simulink library "PlantLibrary"  (R2016b)
settings: Solver=VariableStepAuto  StartTime=0.0  StopTime=10.0  RelTol=1e-3
values from neighbouring files (symbols this model uses):
  amp2mAmp = 1000    [PlantParams.m]
  coilL = 0.125    [PlantParams.m]
  coilMaxI = 0.9*amp2mAmp*Vs/coilR    (= 1800)    [PlantParams.m]
  coilMinI = 0.2*amp2mAmp*Vs/coilR    (= 400)    [PlantParams.m]
  coilR = 6    [PlantParams.m]
  fs = 100    [PlantParams.m]
  maxFlowRate = maxFlowRate*1    (= 16)    [PlantParams.m]
  reducer_ex = 0.01    [PlantParams.m]
  reducer_rt = 0.01    [PlantParams.m]
  strokeLegnth = 500    [PlantParams.m]
  Vs = 12    [PlantParams.m]
undefined symbols (not defined in the file or in its folder): DiscIntNeverNeededParam
undefined symbols (not defined in the file): dampeningFL, extendRateFL, retractRateFL
libraries: PlantLibrary x19, simulink x3, HighClearance_library x1
settings Model: Creator=lemaya  LastModifiedBy=lemaya

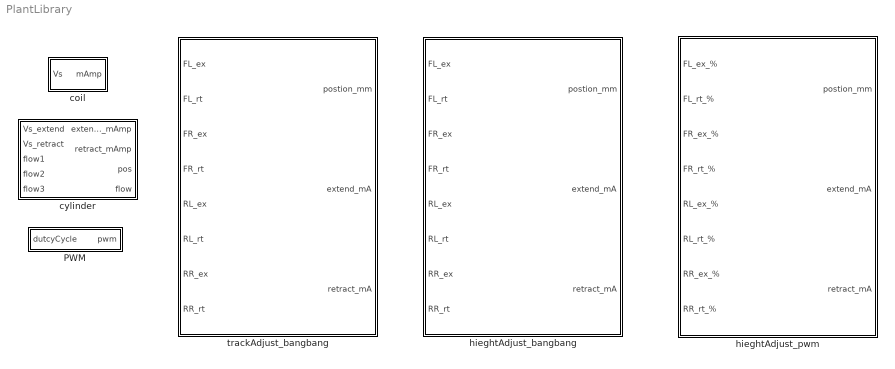
== system PlantLibrary ==
  PWM : Subsystem  TreatAsAtomicUnit=on
  coil : Subsystem
  cylinder : Subsystem  mask{dampening=dampeningFL, extendRate=extendRateFL, retractRate=retractRateFL}
      mask prompts: dampening "Dampening coefficient:"; extendRate "Extend Rate [mm/sec]:"; retractRate "Retract Rate [mm/sec]:"
  hieghtAdjust_bangbang : Subsystem
  hieghtAdjust_pwm : Subsystem
  trackAdjust_bangbang : Subsystem

== system PlantLibrary/PWM ==
  dutcyCycle : Inport
  Data Type Conversion : DataTypeConversion  OutDataTypeStr=single
  Relational Operator : RelationalOperator  Operator=>  OutDataTypeStr=boolean  RndMeth=Simplest
  freq : simulink/Sources/Repeating Sequence  rep_seq_t=[0 1/fs]  rep_seq_y=[0 100]
  pwm : Outport
  wires:
  freq/1 -> Relational Operator/2  "Hz"
  Relational Operator/1 -> Data Type Conversion/1
  dutcyCycle/1 -> Relational Operator/1  "%"
  Data Type Conversion/1 -> pwm/1

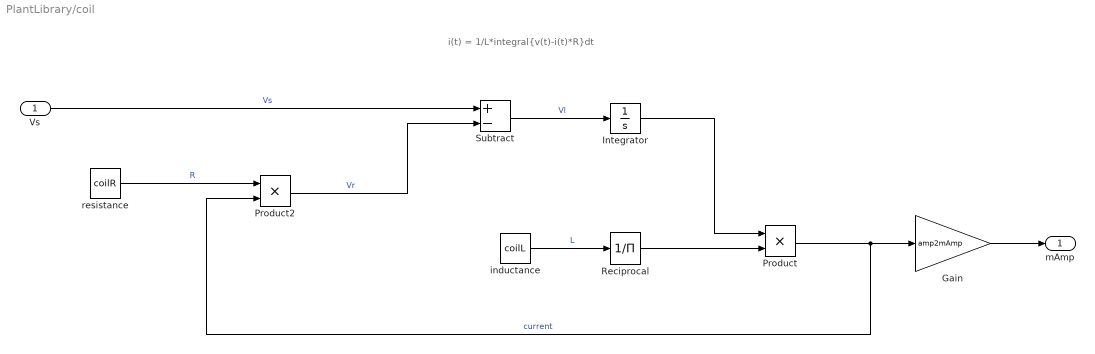
== system PlantLibrary/coil ==
  note: i(t) = 1/L*integral{v(t)-i(t)*R}dt
  Vs : Inport
  Gain : Gain  Gain=amp2mAmp  OutDataTypeStr=single
  Integrator : Integrator
  Product : Product  OutDataTypeStr=single  SaturateOnIntegerOverflow=on
  Product2 : Product  OutDataTypeStr=single  SaturateOnIntegerOverflow=on
  Reciprocal : Product  Inputs=/  SaturateOnIntegerOverflow=on  RndMeth=Zero
  Subtract : Sum  Inputs=+-  OutDataTypeStr=Inherit: Inherit via back propagation  SaturateOnIntegerOverflow=on
  inductance : Constant  Value=coilL  OutDataTypeStr=single
  resistance : Constant  Value=coilR  OutDataTypeStr=single
  mAmp : Outport
  wires:
  Gain/1 -> mAmp/1
  Vs/1 -> Subtract/1  "Vs"
  inductance/1 -> Reciprocal/1  "L"
  Subtract/1 -> Integrator/1  "Vl"
  resistance/1 -> Product2/1  "R"
  Product2/1 -> Subtract/2  "Vr"
  Integrator/1 -> Product/1
  Reciprocal/1 -> Product/2
  Product/1 -> Gain/1, Product2/2  "current"

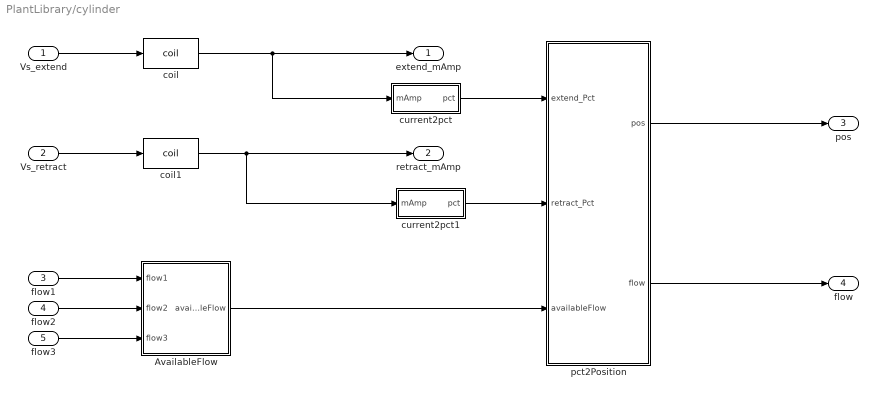
== system PlantLibrary/cylinder ==
  Vs_extend : Inport
  Vs_retract : Inport  Port=2
  flow1 : Inport  Port=3
  flow2 : Inport  Port=4
  flow3 : Inport  Port=5
  AvailableFlow : Subsystem
  coil : PlantLibrary/coil
  coil1 : PlantLibrary/coil
  current2pct : Subsystem
  current2pct1 : Subsystem
  pct2Position : Subsystem
  extend_mAmp : Outport
  retract_mAmp : Outport  Port=2
  pos : Outport  Port=3
  flow : Outport  Port=4
  wires:
  AvailableFlow/1(availableFlow) -> pct2Position/3(availableFlow)
  flow3/1 -> AvailableFlow/3(flow3)
  flow2/1 -> AvailableFlow/2(flow2)
  flow1/1 -> AvailableFlow/1(flow1)
  pct2Position/2(flow) -> flow/1
  pct2Position/1(pos) -> pos/1
  current2pct1/1(pct) -> pct2Position/2(retract_Pct)
  current2pct/1(pct) -> pct2Position/1(extend_Pct)
  coil1/1 -> retract_mAmp/1, current2pct1/1(mAmp)
  coil/1 -> extend_mAmp/1, current2pct/1(mAmp)
  Vs_retract/1 -> coil1/1
  Vs_extend/1 -> coil/1

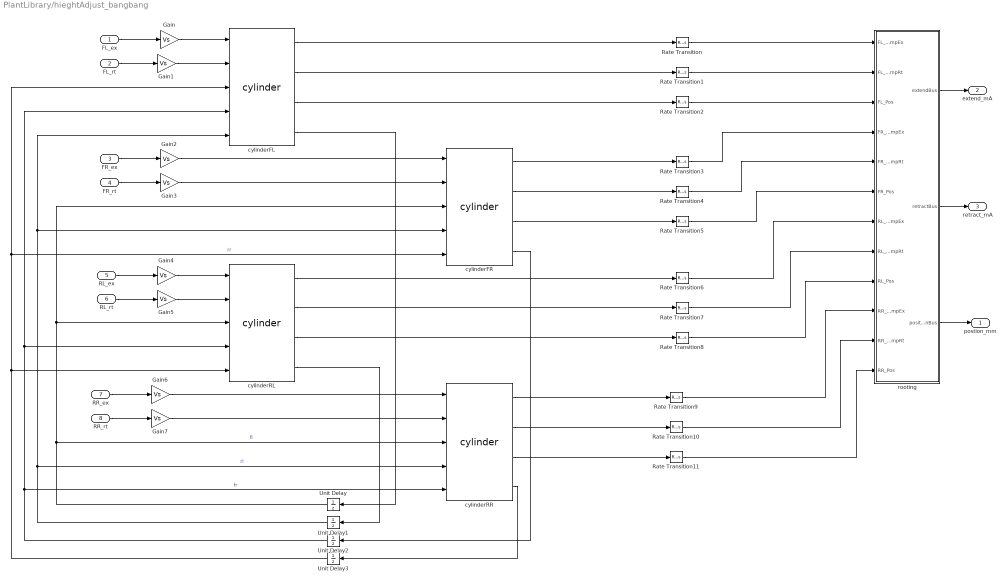
== system PlantLibrary/hieghtAdjust_bangbang ==
  FL_ex : Inport
  FL_rt : Inport  Port=2
  FR_ex : Inport  Port=3
  FR_rt : Inport  Port=4
  RL_ex : Inport  Port=5
  RL_rt : Inport  Port=6
  RR_ex : Inport  Port=7
  RR_rt : Inport  Port=8
  Gain{,1..7} (8 alike) : Gain  Gain=Vs
  Rate Transition{,1..11} (12 alike) : RateTransition
  Unit Delay{,1..3} (4 alike) : UnitDelay  SampleTime=-1
  cylinderFL : PlantLibrary/cylinder  dampening=dampeningFL  extendRate=extendRateFL  retractRate=retractRateFL
  cylinderFR : PlantLibrary/cylinder  dampening=dampeningFR  extendRate=extendRateFR  retractRate=retractRateFR
  cylinderRL : PlantLibrary/cylinder  dampening=dampeningRL  extendRate=extendRateRL  retractRate=retractRateRL
  cylinderRR : PlantLibrary/cylinder  dampening=dampeningRR  extendRate=extendRateRR  retractRate=retractRateRR
  rooting : Subsystem
  postion_mm : Outport
  extend_mA : Outport  Port=2
  retract_mA : Outport  Port=3
  wires:
  Unit Delay/1 -> cylinderRR/3, cylinderRL/3, cylinderFR/3  "fl"
  Unit Delay3/1 -> cylinderFR/5, cylinderFL/3, cylinderRL/5  "rr"
  Unit Delay2/1 -> cylinderRR/5, cylinderRL/4, cylinderFL/4  "fr"
  Unit Delay1/1 -> cylinderRR/4, cylinderFR/4, cylinderFL/5  "rl"
  cylinderRR/4 -> Unit Delay3/1
  cylinderFR/4 -> Unit Delay2/1
  cylinderRL/4 -> Unit Delay1/1
  cylinderFL/4 -> Unit Delay/1
  Gain2/1 -> cylinderFR/1
  Gain3/1 -> cylinderFR/2
  cylinderRR/3 -> Rate Transition11/1
  cylinderFR/3 -> Rate Transition5/1
  cylinderRL/3 -> Rate Transition8/1
  cylinderFL/3 -> Rate Transition2/1
  Rate Transition11/1 -> rooting/12(RR_Pos)
  Rate Transition10/1 -> rooting/11(RR_mAmpRt)
  Rate Transition9/1 -> rooting/10(RR_mAmpEx)
  Rate Transition8/1 -> rooting/9(RL_Pos)
  Rate Transition7/1 -> rooting/8(RL_mAmpRt)
  Rate Transition6/1 -> rooting/7(RL_mAmpEx)
  Rate Transition5/1 -> rooting/6(FR_Pos)
  Rate Transition4/1 -> rooting/5(FR_mAmpRt)
  Rate Transition3/1 -> rooting/4(FR_mAmpEx)
  Rate Transition2/1 -> rooting/3(FL_Pos)
  Rate Transition1/1 -> rooting/2(FL_mAmpRt)
  Rate Transition/1 -> rooting/1(FL_mAmpEx)
  Gain7/1 -> cylinderRR/2
  Gain6/1 -> cylinderRR/1
  Gain5/1 -> cylinderRL/2
  Gain4/1 -> cylinderRL/1
  Gain1/1 -> cylinderFL/2
  Gain/1 -> cylinderFL/1
  RL_rt/1 -> Gain5/1
  RR_ex/1 -> Gain6/1
  FR_rt/1 -> Gain3/1
  FR_ex/1 -> Gain2/1
  FL_ex/1 -> Gain/1
  RL_ex/1 -> Gain4/1
  RR_rt/1 -> Gain7/1
  FL_rt/1 -> Gain1/1
  rooting/1(extendBus) -> extend_mA/1
  rooting/2(retractBus) -> retract_mA/1
  rooting/3(positionBus) -> postion_mm/1
  cylinderFL/1 -> Rate Transition/1
  cylinderFL/2 -> Rate Transition1/1
  cylinderFR/1 -> Rate Transition3/1
  cylinderFR/2 -> Rate Transition4/1
  cylinderRL/1 -> Rate Transition6/1
  cylinderRL/2 -> Rate Transition7/1
  cylinderRR/1 -> Rate Transition9/1
  cylinderRR/2 -> Rate Transition10/1

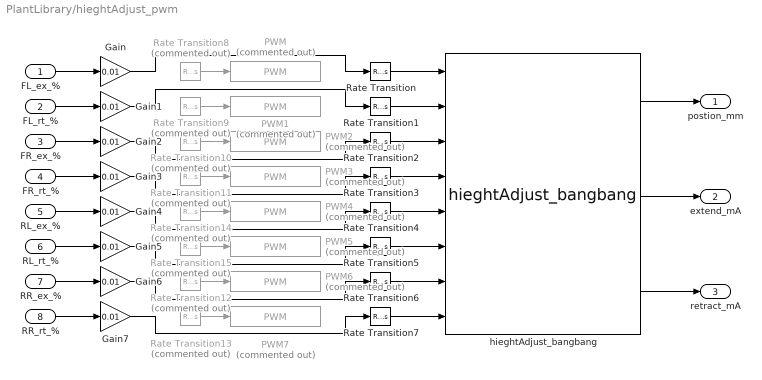
== system PlantLibrary/hieghtAdjust_pwm ==
  FL_ex_% : Inport
  FL_rt_% : Inport  Port=2
  FR_ex_% : Inport  Port=3
  FR_rt_% : Inport  Port=4
  RL_ex_% : Inport  Port=5
  RL_rt_% : Inport  Port=6
  RR_ex_% : Inport  Port=7
  RR_rt_% : Inport  Port=8
  Gain{,1..7} (8 alike) : Gain  Gain=0.01
  PWM{,1..7} (8 alike) : PlantLibrary/PWM  Commented=on
  Rate Transition{,1..7} (8 alike) : RateTransition
  Rate Transition{8..15} (8 alike) : RateTransition  Commented=on  OutPortSampleTime=0.0001
  hieghtAdjust_bangbang : PlantLibrary/hieghtAdjust_bangbang
  postion_mm : Outport
  extend_mA : Outport  Port=2
  retract_mA : Outport  Port=3
  wires:
  Gain7/1 -> Rate Transition7/1
  RR_rt_%/1 -> Gain7/1
  Gain6/1 -> Rate Transition6/1
  RR_ex_%/1 -> Gain6/1
  Gain5/1 -> Rate Transition5/1
  RL_rt_%/1 -> Gain5/1
  Gain4/1 -> Rate Transition4/1
  RL_ex_%/1 -> Gain4/1
  Gain3/1 -> Rate Transition3/1
  FR_rt_%/1 -> Gain3/1
  Gain2/1 -> Rate Transition2/1
  FR_ex_%/1 -> Gain2/1
  Gain/1 -> Rate Transition/1
  Gain1/1 -> Rate Transition1/1
  FL_rt_%/1 -> Gain1/1
  FL_ex_%/1 -> Gain/1
  Rate Transition13/1 -> PWM7/1
  Rate Transition12/1 -> PWM6/1
  Rate Transition15/1 -> PWM5/1
  Rate Transition14/1 -> PWM4/1
  Rate Transition11/1 -> PWM3/1
  Rate Transition10/1 -> PWM2/1
  Rate Transition9/1 -> PWM1/1
  Rate Transition8/1 -> PWM/1
  hieghtAdjust_bangbang/1 -> postion_mm/1
  hieghtAdjust_bangbang/3 -> retract_mA/1
  hieghtAdjust_bangbang/2 -> extend_mA/1
  Rate Transition/1 -> hieghtAdjust_bangbang/1
  Rate Transition1/1 -> hieghtAdjust_bangbang/2
  Rate Transition2/1 -> hieghtAdjust_bangbang/3
  Rate Transition3/1 -> hieghtAdjust_bangbang/4
  Rate Transition4/1 -> hieghtAdjust_bangbang/5
  Rate Transition5/1 -> hieghtAdjust_bangbang/6
  Rate Transition6/1 -> hieghtAdjust_bangbang/7
  Rate Transition7/1 -> hieghtAdjust_bangbang/8

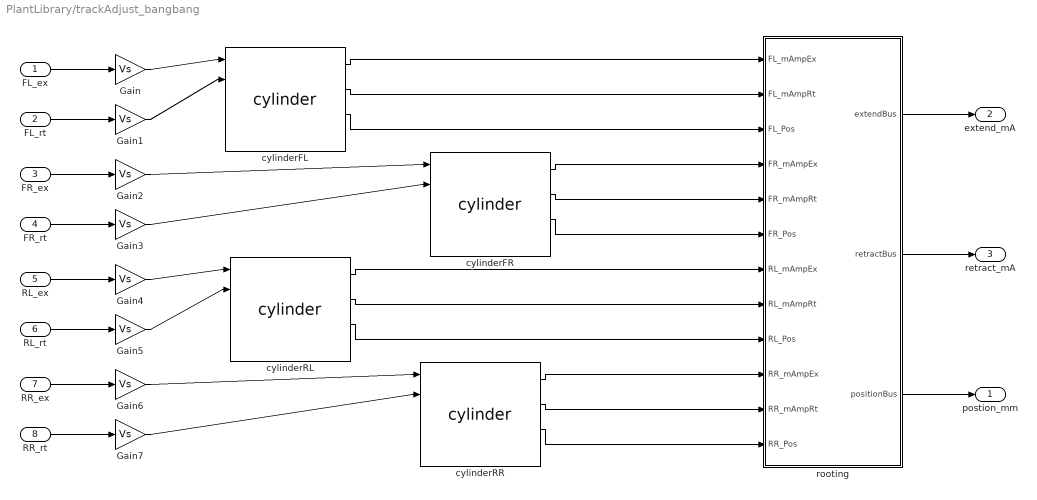
== system PlantLibrary/trackAdjust_bangbang ==
  FL_ex : Inport
  FL_rt : Inport  Port=2
  FR_ex : Inport  Port=3
  FR_rt : Inport  Port=4
  RL_ex : Inport  Port=5
  RL_rt : Inport  Port=6
  RR_ex : Inport  Port=7
  RR_rt : Inport  Port=8
  Gain{,1..7} (8 alike) : Gain  Gain=Vs
  cylinderFL : PlantLibrary/cylinder  dampening=dampening  extendRate=extendRateFL  retractRate=retractRateFL
  cylinderFR : PlantLibrary/cylinder  dampening=dampening  extendRate=extendRateFL  retractRate=retractRateFL
  cylinderRL : PlantLibrary/cylinder  dampening=dampening  extendRate=extendRateFL  retractRate=retractRateFL
  cylinderRR : PlantLibrary/cylinder  dampening=dampening  extendRate=extendRateFL  retractRate=retractRateFL
  rooting : Subsystem
  postion_mm : Outport
  extend_mA : Outport  Port=2
  retract_mA : Outport  Port=3
  wires:
  cylinderRR/3 -> rooting/12(RR_Pos)
  cylinderRR/2 -> rooting/11(RR_mAmpRt)
  cylinderRR/1 -> rooting/10(RR_mAmpEx)
  cylinderRL/3 -> rooting/9(RL_Pos)
  cylinderRL/2 -> rooting/8(RL_mAmpRt)
  cylinderRL/1 -> rooting/7(RL_mAmpEx)
  cylinderFR/3 -> rooting/6(FR_Pos)
  cylinderFR/2 -> rooting/5(FR_mAmpRt)
  cylinderFR/1 -> rooting/4(FR_mAmpEx)
  cylinderFL/3 -> rooting/3(FL_Pos)
  cylinderFL/2 -> rooting/2(FL_mAmpRt)
  cylinderFL/1 -> rooting/1(FL_mAmpEx)
  rooting/3(positionBus) -> postion_mm/1
  rooting/2(retractBus) -> retract_mA/1
  rooting/1(extendBus) -> extend_mA/1
  FL_rt/1 -> Gain1/1
  RR_rt/1 -> Gain7/1
  RL_ex/1 -> Gain4/1
  FL_ex/1 -> Gain/1
  FR_ex/1 -> Gain2/1
  FR_rt/1 -> Gain3/1
  RR_ex/1 -> Gain6/1
  RL_rt/1 -> Gain5/1
  Gain/1 -> cylinderFL/1
  Gain1/1 -> cylinderFL/2
  Gain2/1 -> cylinderFR/1
  Gain3/1 -> cylinderFR/2
  Gain4/1 -> cylinderRL/1
  Gain5/1 -> cylinderRL/2
  Gain6/1 -> cylinderRR/1
  Gain7/1 -> cylinderRR/2

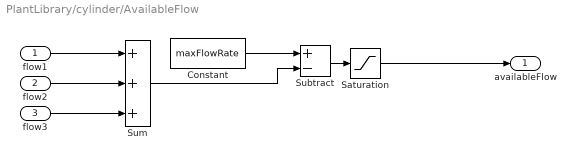
== system PlantLibrary/cylinder/AvailableFlow ==
  flow1 : Inport
  flow2 : Inport  Port=2
  flow3 : Inport  Port=3
  Constant : Constant  Value=maxFlowRate
  Saturation : Saturate  UpperLimit=0  LowerLimit=-inf
  Subtract : Sum  Inputs=+-
  Sum : Sum  Inputs=+++
  availableFlow : Outport
  wires:
  Saturation/1 -> availableFlow/1
  Subtract/1 -> Saturation/1
  Sum/1 -> Subtract/2
  flow2/1 -> Sum/2
  Constant/1 -> Subtract/1
  flow1/1 -> Sum/1
  flow3/1 -> Sum/3

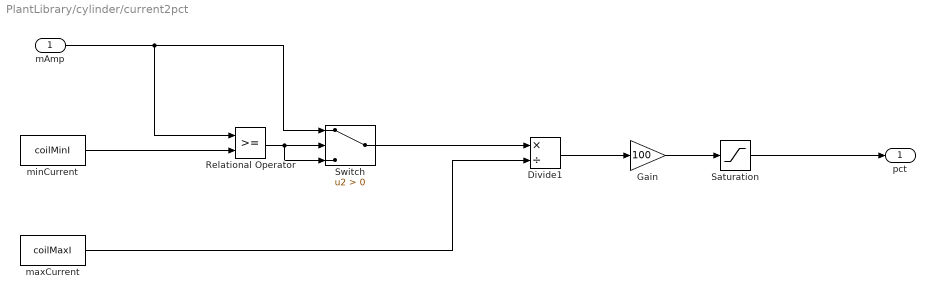
== system PlantLibrary/cylinder/current2pct ==
  mAmp : Inport
  Divide1 : Product  Inputs=*/
  Gain : Gain  Gain=100
  Relational Operator : RelationalOperator  OutDataTypeStr=boolean  RndMeth=Simplest
  Saturation : Saturate  UpperLimit=100  LowerLimit=0
  Switch : Switch  Criteria=u2 > Threshold
  maxCurrent : Constant  Value=coilMaxI
  minCurrent : Constant  Value=coilMinI
  pct : Outport
  wires:
  Gain/1 -> Saturation/1
  Saturation/1 -> pct/1
  Divide1/1 -> Gain/1
  mAmp/1 -> Switch/1, Relational Operator/1
  Switch/1 -> Divide1/1
  minCurrent/1 -> Relational Operator/2
  Relational Operator/1 -> Switch/2, Switch/3
  maxCurrent/1 -> Divide1/2

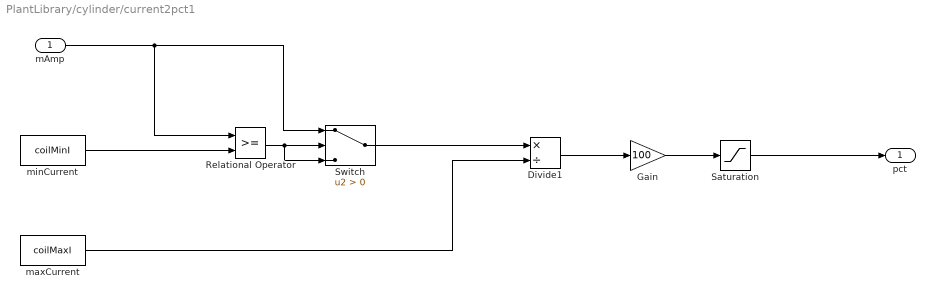
== system PlantLibrary/cylinder/current2pct1 ==
  mAmp : Inport
  Divide1 : Product  Inputs=*/
  Gain : Gain  Gain=100
  Relational Operator : RelationalOperator  OutDataTypeStr=boolean  RndMeth=Simplest
  Saturation : Saturate  UpperLimit=100  LowerLimit=0
  Switch : Switch  Criteria=u2 > Threshold
  maxCurrent : Constant  Value=coilMaxI
  minCurrent : Constant  Value=coilMinI
  pct : Outport
  wires:
  maxCurrent/1 -> Divide1/2
  Relational Operator/1 -> Switch/3, Switch/2
  minCurrent/1 -> Relational Operator/2
  Switch/1 -> Divide1/1
  mAmp/1 -> Relational Operator/1, Switch/1
  Divide1/1 -> Gain/1
  Saturation/1 -> pct/1
  Gain/1 -> Saturation/1

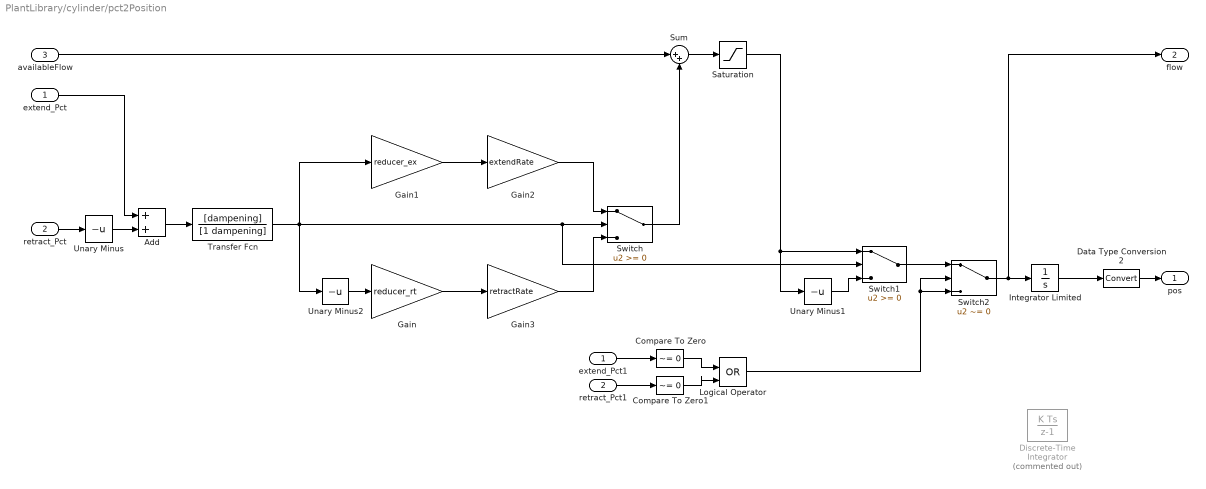
== system PlantLibrary/cylinder/pct2Position ==
  extend_Pct : Inport
  retract_Pct : Inport  Port=2
  availableFlow : Inport  Port=3
  Add : Sum  SaturateOnIntegerOverflow=on
  Compare To Zero : simulink/Logic and Bit Operations/Compare To Zero  relop=~=  OutDataTypeStr=boolean
  Compare To Zero1 : simulink/Logic and Bit Operations/Compare To Zero  relop=~=  OutDataTypeStr=boolean
  Data Type Conversion2 : DataTypeConversion
  Discrete-Time Integrator : DiscreteIntegrator  Commented=on  InitialConditionSetting=State (most efficient)  SampleTime=-1  LimitOutput=on  UpperSaturationLimit=strokeLegnth  LowerSaturationLimit=0  ICPrevOutput=DiscIntNeverNeededParam  ICPrevScaledInput=DiscIntNeverNeededParam
  Gain : Gain  Gain=reducer_rt  OutDataTypeStr=single  SaturateOnIntegerOverflow=on
  Gain1 : Gain  Gain=reducer_ex  OutDataTypeStr=single  SaturateOnIntegerOverflow=on
  Gain2 : Gain  Gain=extendRate  OutDataTypeStr=single  SaturateOnIntegerOverflow=on
  Gain3 : Gain  Gain=retractRate  OutDataTypeStr=single  SaturateOnIntegerOverflow=on
  Integrator Limited : Integrator  LimitOutput=on  UpperSaturationLimit=strokeLegnth  LowerSaturationLimit=0
  Logical Operator : Logic  Operator=OR  IconShape=distinctive  AllPortsSameDT=off  OutDataTypeStr=boolean
  Saturation : Saturate  UpperLimit=inf  LowerLimit=0
  Sum : Sum  Inputs=|++
  Switch : Switch  OutDataTypeStr=Inherit: Inherit via back propagation  SaturateOnIntegerOverflow=on
  Switch1 : Switch  OutDataTypeStr=Inherit: Inherit via back propagation  SaturateOnIntegerOverflow=on
  Switch2 : Switch  Criteria=u2 ~= 0  OutDataTypeStr=Inherit: Inherit via back propagation  SaturateOnIntegerOverflow=on
  Transfer Fcn : TransferFcn  Numerator=[dampening]  Denominator=[1 dampening]
  Unary Minus : UnaryMinus  SaturateOnIntegerOverflow=on
  Unary Minus1 : UnaryMinus  SaturateOnIntegerOverflow=on
  Unary Minus2 : UnaryMinus  SaturateOnIntegerOverflow=on
  extend_Pct1 : InportShadow
  retract_Pct1 : InportShadow  Port=2
  pos : Outport
  flow : Outport  Port=2
  wires:
  Switch2/1 -> flow/1, Integrator Limited/1
  Logical Operator/1 -> Switch2/2, Switch2/3
  Compare To Zero1/1 -> Logical Operator/2
  Compare To Zero/1 -> Logical Operator/1
  retract_Pct1/1 -> Compare To Zero1/1
  extend_Pct1/1 -> Compare To Zero/1
  Saturation/1 -> Switch1/1, Unary Minus1/1
  Unary Minus1/1 -> Switch1/3
  Switch1/1 -> Switch2/1
  Transfer Fcn/1 -> Gain1/1, Unary Minus2/1, Switch1/2, Switch/2
  Unary Minus2/1 -> Gain/1
  Switch/1 -> Sum/2
  availableFlow/1 -> Sum/1
  Integrator Limited/1 -> Data Type Conversion2/1
  Gain3/1 -> Switch/3
  Gain2/1 -> Switch/1
  Sum/1 -> Saturation/1
  Add/1 -> Transfer Fcn/1
  extend_Pct/1 -> Add/1
  Unary Minus/1 -> Add/2
  retract_Pct/1 -> Unary Minus/1
  Data Type Conversion2/1 -> pos/1
  Gain1/1 -> Gain2/1
  Gain/1 -> Gain3/1

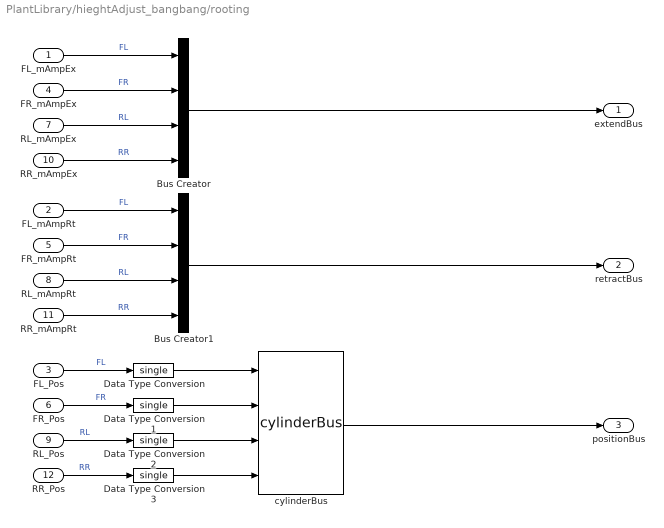
== system PlantLibrary/hieghtAdjust_bangbang/rooting ==
  FL_mAmpEx : Inport
  FL_mAmpRt : Inport  Port=2
  FL_Pos : Inport  Port=3
  FR_mAmpEx : Inport  Port=4
  FR_mAmpRt : Inport  Port=5
  FR_Pos : Inport  Port=6
  RL_mAmpEx : Inport  Port=7
  RL_mAmpRt : Inport  Port=8
  RL_Pos : Inport  Port=9
  RR_mAmpEx : Inport  Port=10
  RR_mAmpRt : Inport  Port=11
  RR_Pos : Inport  Port=12
  Bus Creator : BusCreator  Inputs=4
  Bus Creator1 : BusCreator  Inputs=4
  Data Type Conversion{,1..3} (4 alike) : DataTypeConversion  OutDataTypeStr=single
  cylinderBus : HighClearance_library/cylinderBus
  extendBus : Outport
  retractBus : Outport  Port=2
  positionBus : Outport  Port=3
  wires:
  RR_Pos/1 -> Data Type Conversion3/1  "RR"
  RL_Pos/1 -> Data Type Conversion2/1  "RL"
  FR_Pos/1 -> Data Type Conversion1/1  "FR"
  FL_Pos/1 -> Data Type Conversion/1  "FL"
  Data Type Conversion3/1 -> cylinderBus/4
  Data Type Conversion2/1 -> cylinderBus/3
  Data Type Conversion1/1 -> cylinderBus/2
  Data Type Conversion/1 -> cylinderBus/1
  cylinderBus/1 -> positionBus/1
  FL_mAmpEx/1 -> Bus Creator/1  "FL"
  FR_mAmpEx/1 -> Bus Creator/2  "FR"
  RL_mAmpEx/1 -> Bus Creator/3  "RL"
  RR_mAmpEx/1 -> Bus Creator/4  "RR"
  FL_mAmpRt/1 -> Bus Creator1/1  "FL"
  FR_mAmpRt/1 -> Bus Creator1/2  "FR"
  RL_mAmpRt/1 -> Bus Creator1/3  "RL"
  RR_mAmpRt/1 -> Bus Creator1/4  "RR"
  Bus Creator/1 -> extendBus/1
  Bus Creator1/1 -> retractBus/1

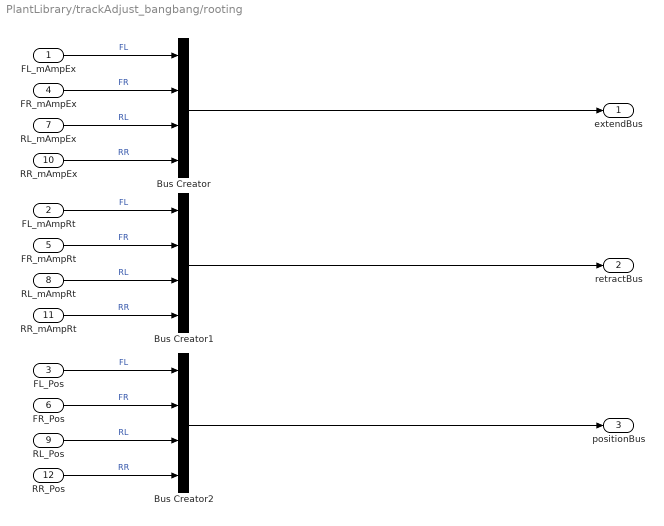
== system PlantLibrary/trackAdjust_bangbang/rooting ==
  FL_mAmpEx : Inport
  FL_mAmpRt : Inport  Port=2
  FL_Pos : Inport  Port=3
  FR_mAmpEx : Inport  Port=4
  FR_mAmpRt : Inport  Port=5
  FR_Pos : Inport  Port=6
  RL_mAmpEx : Inport  Port=7
  RL_mAmpRt : Inport  Port=8
  RL_Pos : Inport  Port=9
  RR_mAmpEx : Inport  Port=10
  RR_mAmpRt : Inport  Port=11
  RR_Pos : Inport  Port=12
  Bus Creator : BusCreator  Inputs=4
  Bus Creator1 : BusCreator  Inputs=4
  Bus Creator2 : BusCreator  Inputs=4
  extendBus : Outport
  retractBus : Outport  Port=2
  positionBus : Outport  Port=3
  wires:
  Bus Creator2/1 -> positionBus/1
  Bus Creator1/1 -> retractBus/1
  Bus Creator/1 -> extendBus/1
  RR_Pos/1 -> Bus Creator2/4  "RR"
  RL_Pos/1 -> Bus Creator2/3  "RL"
  FR_Pos/1 -> Bus Creator2/2  "FR"
  FL_Pos/1 -> Bus Creator2/1  "FL"
  RR_mAmpRt/1 -> Bus Creator1/4  "RR"
  RL_mAmpRt/1 -> Bus Creator1/3  "RL"
  FR_mAmpRt/1 -> Bus Creator1/2  "FR"
  FL_mAmpRt/1 -> Bus Creator1/1  "FL"
  RR_mAmpEx/1 -> Bus Creator/4  "RR"
  RL_mAmpEx/1 -> Bus Creator/3  "RL"
  FR_mAmpEx/1 -> Bus Creator/2  "FR"
  FL_mAmpEx/1 -> Bus Creator/1  "FL"
